simulink model "platooning_multiple_followers"  (R2018a)
settings: Solver=FixedStepAuto  StartTime=0.0  StopTime=70  FixedStep=timestep  RelTol=1e-3
model workspace (MAT data in the model file):
  t_0 = 0
undefined symbols (not defined in the file): a_max, a_min, canChannel, follower_1, follower_2, follower_3, leader, N
libraries: canlib x16, canmsglib x15, dspstat3 x3, dspindex x3, simulink x1
(part 2 of 2)

== system platooning_multiple_followers/speed_check/If Action Subsystem1 ==
  time : Inport
  velocity : Inport  Port=2
  position : Inport  Port=3
  Action Port : ActionPort  ActionType=then
  CAN Pack : canmsglib/CAN Pack  MsgList=(none)  MsgName=CAN Msg  MsgIDType=Standard (11-bit identifier)  MsgIdentifier=1  MsgLength=8  SignalInfo=position$0$16$1$1$1$0$0.1$0$-Inf$Inf$#velocity$16$16$1$1$1$0$0.0025$0$-Inf$Inf$#timestamp$32$16$1$1$1$0$0.01$0$-Inf$Inf$#  NSignals=3  StartBits=str2num('[int32(0);int32(16);int32(32)]')  SignalSizes=str2num('[int32(16);int32(16);int32(16)]')  ByteOrders=str2num('[int32(1);int32(1);int32(1)]')  DataTypes=str2num('[int32(1);int32(1);int32(1)]')  MultiplexTypes=str2num('[int32(1);int32(1);int32(1)]')  MultiplexValues=str2num('[double(0);double(0);double(0)]')  Factors=str2num('[double(0.1);double(0.0025);double(0.01)]')  Offsets=str2num('[double(0);double(0);double(0)]')  Minimums=str2num('[double(-Inf);double(-Inf);double(-Inf)]')  Maximums=str2num('[double(Inf);double(Inf);double(Inf)]')  Remote=off  ApplyMinMax=off
      settings: SourceProductName=Simulink Real-Time  DataFormat=manually specified signals
  CAN Transmit : canlib/CAN Transmit  BlockHandle=784.0001  DeviceMenu=MathWorks Virtual 1 (Channel 1)  Device=MathWorks Virtual 1 (Channel 1)  ObjConstructor=canChannel('MathWorks','Virtual 1',1)  EnablePeriodicTransmit=off  MessagePeriod=1.000
      settings: SourceProductName=Vehicle Network Toolbox  SourceProductBaseCode=VN
  Data Store Write : DataStoreWrite  DataStoreName=t1
  Data Store Write1 : DataStoreWrite  DataStoreName=v1
  Data Store Write2 : DataStoreWrite  DataStoreName=x1
  wires:
  time/1 -> CAN Pack/3, Data Store Write/1
  velocity/1 -> CAN Pack/2, Data Store Write1/1
  CAN Pack/1 -> CAN Transmit/1
  position/1 -> Data Store Write2/1, CAN Pack/1

== system platooning_multiple_followers/speed_check1/If Action Subsystem1 ==
  time : Inport
  velocity : Inport  Port=2
  position : Inport  Port=3
  Action Port : ActionPort  ActionType=then
  CAN Pack : canmsglib/CAN Pack  MsgList=(none)  MsgName=CAN Msg  MsgIDType=Standard (11-bit identifier)  MsgIdentifier=2  MsgLength=8  SignalInfo=position$0$16$1$1$1$0$0.1$0$-Inf$Inf$#velocity$16$16$1$1$1$0$0.0025$0$-Inf$Inf$#timestamp$32$16$1$1$1$0$0.01$0$-Inf$Inf$#  NSignals=3  StartBits=str2num('[int32(0);int32(16);int32(32)]')  SignalSizes=str2num('[int32(16);int32(16);int32(16)]')  ByteOrders=str2num('[int32(1);int32(1);int32(1)]')  DataTypes=str2num('[int32(1);int32(1);int32(1)]')  MultiplexTypes=str2num('[int32(1);int32(1);int32(1)]')  MultiplexValues=str2num('[double(0);double(0);double(0)]')  Factors=str2num('[double(0.1);double(0.0025);double(0.01)]')  Offsets=str2num('[double(0);double(0);double(0)]')  Minimums=str2num('[double(-Inf);double(-Inf);double(-Inf)]')  Maximums=str2num('[double(Inf);double(Inf);double(Inf)]')  Remote=off  ApplyMinMax=off
      settings: SourceProductName=Simulink Real-Time  DataFormat=manually specified signals
  CAN Transmit : canlib/CAN Transmit  BlockHandle=825.0001  DeviceMenu=MathWorks Virtual 1 (Channel 1)  Device=MathWorks Virtual 1 (Channel 1)  ObjConstructor=canChannel('MathWorks','Virtual 1',1)  EnablePeriodicTransmit=off  MessagePeriod=1.000
      settings: SourceProductName=Vehicle Network Toolbox  SourceProductBaseCode=VN
  Data Store Write : DataStoreWrite  DataStoreName=t2
  Data Store Write1 : DataStoreWrite  DataStoreName=t2
  Data Store Write2 : DataStoreWrite  DataStoreName=x2
  wires:
  time/1 -> CAN Pack/3, Data Store Write/1
  velocity/1 -> CAN Pack/2, Data Store Write1/1
  CAN Pack/1 -> CAN Transmit/1
  position/1 -> Data Store Write2/1, CAN Pack/1

== system platooning_multiple_followers/speed_check2/If Action Subsystem1 ==
  time : Inport
  velocity : Inport  Port=2
  position : Inport  Port=3
  Action Port : ActionPort  ActionType=then
  CAN Pack : canmsglib/CAN Pack  MsgList=(none)  MsgName=CAN Msg  MsgIDType=Standard (11-bit identifier)  MsgIdentifier=3  MsgLength=8  SignalInfo=position$0$16$1$1$1$0$0.1$0$-Inf$Inf$#velocity$16$16$1$1$1$0$0.0025$0$-Inf$Inf$#timestamp$32$16$1$1$1$0$0.01$0$-Inf$Inf$#  NSignals=3  StartBits=str2num('[int32(0);int32(16);int32(32)]')  SignalSizes=str2num('[int32(16);int32(16);int32(16)]')  ByteOrders=str2num('[int32(1);int32(1);int32(1)]')  DataTypes=str2num('[int32(1);int32(1);int32(1)]')  MultiplexTypes=str2num('[int32(1);int32(1);int32(1)]')  MultiplexValues=str2num('[double(0);double(0);double(0)]')  Factors=str2num('[double(0.1);double(0.0025);double(0.01)]')  Offsets=str2num('[double(0);double(0);double(0)]')  Minimums=str2num('[double(-Inf);double(-Inf);double(-Inf)]')  Maximums=str2num('[double(Inf);double(Inf);double(Inf)]')  Remote=off  ApplyMinMax=off
      settings: SourceProductName=Simulink Real-Time  DataFormat=manually specified signals
  CAN Transmit : canlib/CAN Transmit  BlockHandle=866.0001  DeviceMenu=MathWorks Virtual 1 (Channel 1)  Device=MathWorks Virtual 1 (Channel 1)  ObjConstructor=canChannel('MathWorks','Virtual 1',1)  EnablePeriodicTransmit=off  MessagePeriod=1.000
      settings: SourceProductName=Vehicle Network Toolbox  SourceProductBaseCode=VN
  Data Store Write : DataStoreWrite  DataStoreName=t3
  Data Store Write1 : DataStoreWrite  DataStoreName=t3
  Data Store Write2 : DataStoreWrite  DataStoreName=x3
  wires:
  time/1 -> CAN Pack/3, Data Store Write/1
  velocity/1 -> CAN Pack/2, Data Store Write1/1
  CAN Pack/1 -> CAN Transmit/1
  position/1 -> Data Store Write2/1, CAN Pack/1

== system platooning_multiple_followers/speed_check3/If Action Subsystem1 ==
  time : Inport
  velocity : Inport  Port=2
  position : Inport  Port=3
  Action Port : ActionPort  ActionType=then
  CAN Pack : canmsglib/CAN Pack  MsgList=(none)  MsgName=CAN Msg  MsgIDType=Standard (11-bit identifier)  MsgIdentifier=4  MsgLength=8  SignalInfo=position$0$16$1$1$1$0$0.1$0$-Inf$Inf$#velocity$16$16$1$1$1$0$0.0025$0$-Inf$Inf$#timestamp$32$16$1$1$1$0$0.01$0$-Inf$Inf$#  NSignals=3  StartBits=str2num('[int32(0);int32(16);int32(32)]')  SignalSizes=str2num('[int32(16);int32(16);int32(16)]')  ByteOrders=str2num('[int32(1);int32(1);int32(1)]')  DataTypes=str2num('[int32(1);int32(1);int32(1)]')  MultiplexTypes=str2num('[int32(1);int32(1);int32(1)]')  MultiplexValues=str2num('[double(0);double(0);double(0)]')  Factors=str2num('[double(0.1);double(0.0025);double(0.01)]')  Offsets=str2num('[double(0);double(0);double(0)]')  Minimums=str2num('[double(-Inf);double(-Inf);double(-Inf)]')  Maximums=str2num('[double(Inf);double(Inf);double(Inf)]')  Remote=off  ApplyMinMax=off
      settings: SourceProductName=Simulink Real-Time  DataFormat=manually specified signals
  CAN Transmit : canlib/CAN Transmit  BlockHandle=907.0001  DeviceMenu=MathWorks Virtual 1 (Channel 1)  Device=MathWorks Virtual 1 (Channel 1)  ObjConstructor=canChannel('MathWorks','Virtual 1',1)  EnablePeriodicTransmit=off  MessagePeriod=1.000
      settings: SourceProductName=Vehicle Network Toolbox  SourceProductBaseCode=VN
  Data Store Write : DataStoreWrite  DataStoreName=t4
  Data Store Write1 : DataStoreWrite  DataStoreName=t4
  Data Store Write2 : DataStoreWrite  DataStoreName=x4
  wires:
  time/1 -> CAN Pack/3, Data Store Write/1
  velocity/1 -> CAN Pack/2, Data Store Write1/1
  CAN Pack/1 -> CAN Transmit/1
  position/1 -> Data Store Write2/1, CAN Pack/1

== system platooning_multiple_followers/time_check/If Action Subsystem ==
  time : Inport
  velocity : Inport  Port=2
  position : Inport  Port=3
  Action Port : ActionPort  ActionType=then
  CAN Pack : canmsglib/CAN Pack  MsgList=(none)  MsgName=CAN Msg  MsgIDType=Standard (11-bit identifier)  MsgIdentifier=1  MsgLength=8  SignalInfo=position$0$16$1$1$1$0$0.1$0$-Inf$Inf$#velocity$16$16$1$1$1$0$0.0025$0$-Inf$Inf$#timestamp$32$16$1$1$1$0$0.01$0$-Inf$Inf$#  NSignals=3  StartBits=str2num('[int32(0);int32(16);int32(32)]')  SignalSizes=str2num('[int32(16);int32(16);int32(16)]')  ByteOrders=str2num('[int32(1);int32(1);int32(1)]')  DataTypes=str2num('[int32(1);int32(1);int32(1)]')  MultiplexTypes=str2num('[int32(1);int32(1);int32(1)]')  MultiplexValues=str2num('[double(0);double(0);double(0)]')  Factors=str2num('[double(0.1);double(0.0025);double(0.01)]')  Offsets=str2num('[double(0);double(0);double(0)]')  Minimums=str2num('[double(-Inf);double(-Inf);double(-Inf)]')  Maximums=str2num('[double(Inf);double(Inf);double(Inf)]')  Remote=off  ApplyMinMax=off
      settings: SourceProductName=Simulink Real-Time  DataFormat=manually specified signals
  CAN Transmit : canlib/CAN Transmit  BlockHandle=947.0001  DeviceMenu=MathWorks Virtual 1 (Channel 1)  Device=MathWorks Virtual 1 (Channel 1)  ObjConstructor=canChannel('MathWorks','Virtual 1',1)  EnablePeriodicTransmit=off  MessagePeriod=1.000
      settings: SourceProductName=Vehicle Network Toolbox  SourceProductBaseCode=VN
  Data Store Write : DataStoreWrite  DataStoreName=t1
  Data Store Write1 : DataStoreWrite  DataStoreName=v1
  Data Store Write2 : DataStoreWrite  DataStoreName=x1
  wires:
  time/1 -> CAN Pack/3, Data Store Write/1
  velocity/1 -> CAN Pack/2, Data Store Write1/1
  CAN Pack/1 -> CAN Transmit/1
  position/1 -> Data Store Write2/1, CAN Pack/1

== system platooning_multiple_followers/time_check1/If Action Subsystem ==
  time : Inport
  velocity : Inport  Port=2
  position : Inport  Port=3
  Action Port : ActionPort  ActionType=then
  CAN Pack : canmsglib/CAN Pack  MsgList=(none)  MsgName=CAN Msg  MsgIDType=Standard (11-bit identifier)  MsgIdentifier=2  MsgLength=8  SignalInfo=position$0$16$1$1$1$0$0.1$0$-Inf$Inf$#velocity$16$16$1$1$1$0$0.0025$0$-Inf$Inf$#timestamp$32$16$1$1$1$0$0.01$0$-Inf$Inf$#  NSignals=3  StartBits=str2num('[int32(0);int32(16);int32(32)]')  SignalSizes=str2num('[int32(16);int32(16);int32(16)]')  ByteOrders=str2num('[int32(1);int32(1);int32(1)]')  DataTypes=str2num('[int32(1);int32(1);int32(1)]')  MultiplexTypes=str2num('[int32(1);int32(1);int32(1)]')  MultiplexValues=str2num('[double(0);double(0);double(0)]')  Factors=str2num('[double(0.1);double(0.0025);double(0.01)]')  Offsets=str2num('[double(0);double(0);double(0)]')  Minimums=str2num('[double(-Inf);double(-Inf);double(-Inf)]')  Maximums=str2num('[double(Inf);double(Inf);double(Inf)]')  Remote=off  ApplyMinMax=off
      settings: SourceProductName=Simulink Real-Time  DataFormat=manually specified signals
  CAN Transmit : canlib/CAN Transmit  BlockHandle=978.0001  DeviceMenu=MathWorks Virtual 1 (Channel 1)  Device=MathWorks Virtual 1 (Channel 1)  ObjConstructor=canChannel('MathWorks','Virtual 1',1)  EnablePeriodicTransmit=off  MessagePeriod=1.000
      settings: SourceProductName=Vehicle Network Toolbox  SourceProductBaseCode=VN
  Data Store Write : DataStoreWrite  DataStoreName=t2
  Data Store Write1 : DataStoreWrite  DataStoreName=v2
  Data Store Write2 : DataStoreWrite  DataStoreName=x2
  wires:
  time/1 -> CAN Pack/3, Data Store Write/1
  velocity/1 -> CAN Pack/2, Data Store Write1/1
  CAN Pack/1 -> CAN Transmit/1
  position/1 -> Data Store Write2/1, CAN Pack/1

== system platooning_multiple_followers/time_check2/If Action Subsystem ==
  time : Inport
  velocity : Inport  Port=2
  position : Inport  Port=3
  Action Port : ActionPort  ActionType=then
  CAN Pack : canmsglib/CAN Pack  MsgList=(none)  MsgName=CAN Msg  MsgIDType=Standard (11-bit identifier)  MsgIdentifier=3  MsgLength=8  SignalInfo=position$0$16$1$1$1$0$0.1$0$-Inf$Inf$#velocity$16$16$1$1$1$0$0.0025$0$-Inf$Inf$#timestamp$32$16$1$1$1$0$0.01$0$-Inf$Inf$#  NSignals=3  StartBits=str2num('[int32(0);int32(16);int32(32)]')  SignalSizes=str2num('[int32(16);int32(16);int32(16)]')  ByteOrders=str2num('[int32(1);int32(1);int32(1)]')  DataTypes=str2num('[int32(1);int32(1);int32(1)]')  MultiplexTypes=str2num('[int32(1);int32(1);int32(1)]')  MultiplexValues=str2num('[double(0);double(0);double(0)]')  Factors=str2num('[double(0.1);double(0.0025);double(0.01)]')  Offsets=str2num('[double(0);double(0);double(0)]')  Minimums=str2num('[double(-Inf);double(-Inf);double(-Inf)]')  Maximums=str2num('[double(Inf);double(Inf);double(Inf)]')  Remote=off  ApplyMinMax=off
      settings: SourceProductName=Simulink Real-Time  DataFormat=manually specified signals
  CAN Transmit : canlib/CAN Transmit  BlockHandle=1009.0001  DeviceMenu=MathWorks Virtual 1 (Channel 1)  Device=MathWorks Virtual 1 (Channel 1)  ObjConstructor=canChannel('MathWorks','Virtual 1',1)  EnablePeriodicTransmit=off  MessagePeriod=1.000
      settings: SourceProductName=Vehicle Network Toolbox  SourceProductBaseCode=VN
  Data Store Write : DataStoreWrite  DataStoreName=t3
  Data Store Write1 : DataStoreWrite  DataStoreName=v3
  Data Store Write2 : DataStoreWrite  DataStoreName=x3
  wires:
  time/1 -> CAN Pack/3, Data Store Write/1
  velocity/1 -> CAN Pack/2, Data Store Write1/1
  CAN Pack/1 -> CAN Transmit/1
  position/1 -> Data Store Write2/1, CAN Pack/1

== system platooning_multiple_followers/time_check3/If Action Subsystem ==
  time : Inport
  velocity : Inport  Port=2
  position : Inport  Port=3
  Action Port : ActionPort  ActionType=then
  CAN Pack : canmsglib/CAN Pack  MsgList=(none)  MsgName=CAN Msg  MsgIDType=Standard (11-bit identifier)  MsgIdentifier=4  MsgLength=8  SignalInfo=position$0$16$1$1$1$0$0.1$0$-Inf$Inf$#velocity$16$16$1$1$1$0$0.0025$0$-Inf$Inf$#timestamp$32$16$1$1$1$0$0.01$0$-Inf$Inf$#  NSignals=3  StartBits=str2num('[int32(0);int32(16);int32(32)]')  SignalSizes=str2num('[int32(16);int32(16);int32(16)]')  ByteOrders=str2num('[int32(1);int32(1);int32(1)]')  DataTypes=str2num('[int32(1);int32(1);int32(1)]')  MultiplexTypes=str2num('[int32(1);int32(1);int32(1)]')  MultiplexValues=str2num('[double(0);double(0);double(0)]')  Factors=str2num('[double(0.1);double(0.0025);double(0.01)]')  Offsets=str2num('[double(0);double(0);double(0)]')  Minimums=str2num('[double(-Inf);double(-Inf);double(-Inf)]')  Maximums=str2num('[double(Inf);double(Inf);double(Inf)]')  Remote=off  ApplyMinMax=off
      settings: SourceProductName=Simulink Real-Time  DataFormat=manually specified signals
  CAN Transmit : canlib/CAN Transmit  BlockHandle=1040.0004  DeviceMenu=MathWorks Virtual 1 (Channel 1)  Device=MathWorks Virtual 1 (Channel 1)  ObjConstructor=canChannel('MathWorks','Virtual 1',1)  EnablePeriodicTransmit=off  MessagePeriod=1.000
      settings: SourceProductName=Vehicle Network Toolbox  SourceProductBaseCode=VN
  Data Store Write : DataStoreWrite  DataStoreName=t4
  Data Store Write1 : DataStoreWrite  DataStoreName=v4
  Data Store Write2 : DataStoreWrite  DataStoreName=x4
  wires:
  time/1 -> CAN Pack/3, Data Store Write/1
  velocity/1 -> CAN Pack/2, Data Store Write1/1
  CAN Pack/1 -> CAN Transmit/1
  position/1 -> Data Store Write2/1, CAN Pack/1
